simulink model "dynamic_model_v4"  (R2022a)
settings: Solver=VariableStepAuto  StartTime=0.0  StopTime=T  FixedStep=0.001  RelTol=1e-3  AbsTol=1e-3  EnableMultiTasking=on
values from neighbouring files (symbols this model uses):
  Kv = 1*(ones(3,3))    [RBT_UR5_NN_adaptation.m]    (also in dynamic_model_code.m = [1.5, 0, 0)
  lamda = 0.1    [RBT_UR5_NN_adaptation.m]    (also in dynamic_model_code.m = 1.2)
  M = A1*layer1    [M_cap.m]    (also in dynamic_model_code.m = 5)
  m1 = 1    [dynamic_model_code.m]
  m2 = 0.5    [dynamic_model_code.m]
  m3 = 0.25    [dynamic_model_code.m]
  s = tf('s')    [tf_compute.m]
  w = zeros(3,1)    [RBT_UR5_NN_adaptation.m]    (also in dynamic_model_code.m)
undefined symbols (not defined in the file or in its folder): X, Y, Z
libraries: sm_lib x15, nesl_utility x13, simulink x9
settings Model: Creator=khan  LastModifiedBy=khan
settings SolverCC: AutoScaleAbsTol=off  AlgebraicLoopSolver=TrustRegion  MaxZcPerStep=1
settings DataIOCC: LimitDataPoints=on  MaxDataPoints=10000
settings OptimizationCC: LifeSpan=inf
settings DebuggingCC: UnconnectedInputMsg=warning  UnconnectedOutputMsg=warning  UnconnectedLineMsg=warning  AllowSymbolicDim=off  SFUnexpectedBacktrackingDiag=warning  SFNoUnconditionalDefaultTransitionDiag=warning  SFExecutionAtInitializationDiag=none  SFMachineParentedDataDiag=warning  ArithmeticOperatorsInVariantConditions=warning
settings SFSimCC: SimUseLocalCustomCode=off  CustomCodeUndefinedFunction=UseInterfaceOnly
settings RTWCC: RTWUseLocalCustomCode=off  DLArmComputeVersion=19.05
settings CodeAppCC: StateflowObjectComments=on
settings GRTTargetCC: TargetLangStandard=C89/C90 (ANSI)
settings ConfigComp: CovMetricSettings=dw  CovSaveCumulativeToWorkspaceVar=on  CovSaveSingleToWorkspaceVar=on  CovExternalEMLEnable=off  CovSFcnEnable=off
settings SimscapeCC: SimscapeLogType=all  SimscapeLogSimulationStatistics=on  SimscapeLogDataHistory=10000

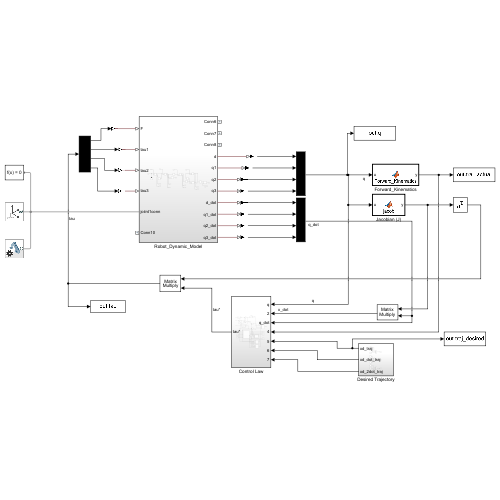
[thumbnail: Simulink's stored preview of the top-level diagram]
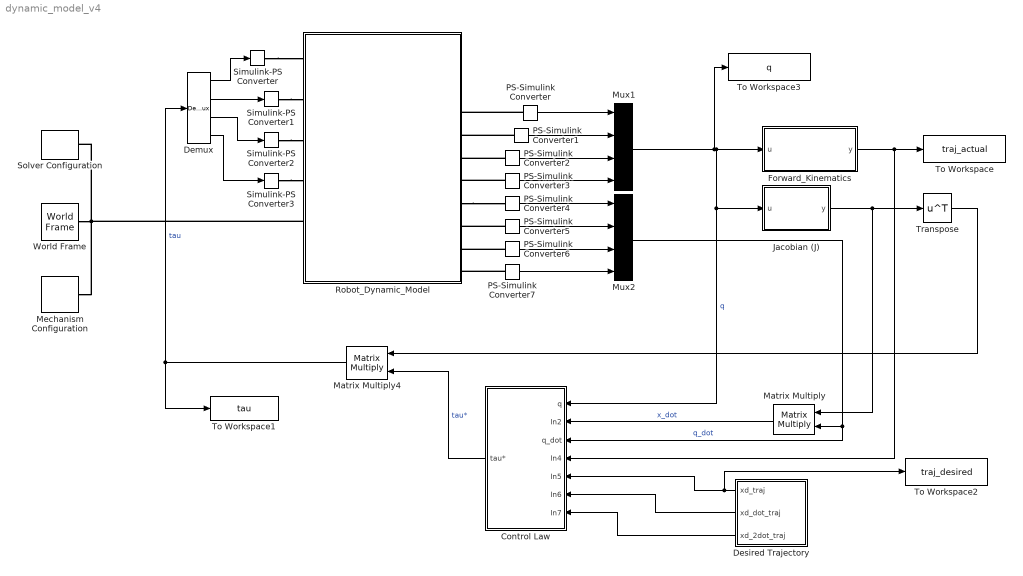
== system dynamic_model_v4 ==
  Control Law : Subsystem
  Demux : Demux
  Desired Trajectory : Subsystem
  Forward_Kinematics : MATLAB Function  TreatAsAtomicUnit=on
  Jacobian (J) : MATLAB Function  TreatAsAtomicUnit=on
  Matrix Multiply : Product  Multiplication=Matrix(*)
  Matrix Multiply4 : Product  Multiplication=Matrix(*)
  Mechanism Configuration : sm_lib/Utilities/Mechanism Configuration  UniformGravity=Constant  GravityVector=[0 0 -9.80665]  GravityUnits=m/s^2  LinearizationDelta=0.001  JointModeTransitionNonlinearIterations=2
  Mux1 : Mux
  Mux2 : Mux
  PS-Simulink Converter{,1..7} (8 alike) : nesl_utility/PS-Simulink Converter  PhysicalDomain=network_engine_domain  SubClassName=ps_output  LeftPortType=input  RightPortType=output  PseudoPeriodic=off  Frequencies=[]  VectorFormat=inherit  Unit=inherit  AffineConversion=off
      settings: SourceProductBaseCode=SS,PW,VE
  Robot_Dynamic_Model : Subsystem
  Simulink-PS Converter : nesl_utility/Simulink-PS Converter  PhysicalDomain=network_engine_domain  SubClassName=ps_input  LeftPortType=input  RightPortType=output  PseudoPeriodic=off  Frequencies=[]  NoiseDistribution=none  NoiseParameters=[]  Unit=N  AffineConversion=off  FilteringAndDerivatives=provide  SimscapeFilterOrder=1  InputFilterTimeConstant=0.001  UdotUserProvided=0
      settings: SourceProductBaseCode=SS,PW,VE
  Simulink-PS Converter1 : nesl_utility/Simulink-PS Converter  PhysicalDomain=network_engine_domain  SubClassName=ps_input  LeftPortType=input  RightPortType=output  PseudoPeriodic=off  Frequencies=[]  NoiseDistribution=none  NoiseParameters=[]  Unit=N*m  AffineConversion=off  FilteringAndDerivatives=provide  SimscapeFilterOrder=1  InputFilterTimeConstant=0.001  UdotUserProvided=0
      settings: SourceProductBaseCode=SS,PW,VE
  Simulink-PS Converter2 : nesl_utility/Simulink-PS Converter  PhysicalDomain=network_engine_domain  SubClassName=ps_input  LeftPortType=input  RightPortType=output  PseudoPeriodic=off  Frequencies=[]  NoiseDistribution=none  NoiseParameters=[]  Unit=N*m  AffineConversion=off  FilteringAndDerivatives=provide  SimscapeFilterOrder=1  InputFilterTimeConstant=0.001  UdotUserProvided=0
      settings: SourceProductBaseCode=SS,PW,VE
  Simulink-PS Converter3 : nesl_utility/Simulink-PS Converter  PhysicalDomain=network_engine_domain  SubClassName=ps_input  LeftPortType=input  RightPortType=output  PseudoPeriodic=off  Frequencies=[]  NoiseDistribution=none  NoiseParameters=[]  Unit=N*m  AffineConversion=off  FilteringAndDerivatives=provide  SimscapeFilterOrder=1  InputFilterTimeConstant=0.001  UdotUserProvided=0
      settings: SourceProductBaseCode=SS,PW,VE
  Solver Configuration : nesl_utility/Solver Configuration  PhysicalDomain=network_engine_domain  SubClassName=solver  LeftPortType=input  RightPortType=generic  Tones=[]  Harmonics=[]  SimulateNoise=off  Profile=off  UseLocalSampling=off  EnableSwitchedLinearOptims=on  FrequencyDomain=off  UseCCode=off  RelTol=0.001  AbsTol=1e-06  MinStep=1e-09  ToWorkspace=off  RevertToSquareIcSolve=off  NumHomotopyIterations=100  PhasorMode=off  PhasorModeNumHarmonics=1  IndexReductionMethod=DerivativeReplacement  DoDC=off  ResidualTolerance=1e-09  UseLocalSolver=off  LocalSolverChoice=NE_BACKWARD_EULER_ADVANCER  LocalSolverSampleTime=0.001  DoFixedCost=off  MaxNonlinIter=3  MaxModeIter=2  ComputeImpulses=off  ImpulseIterations=2  LinearAlgebra=Sparse  LinearAlgebraNumThread=0  EquationFormulation=NE_TIME_EF  DelaysMemoryBudget=1024  AutomaticFiltering=on  FilteringTimeConstant=0.001  PartitionStorageMethod=AS_NEEDED  PartitionMemoryBudget=1024  PartitionMethod=FAST
      settings: SourceProductBaseCode=SS,PW,VE
  To Workspace : ToWorkspace  VariableName=traj_actual  SampleTime=-1
  To Workspace1 : ToWorkspace  VariableName=tau  SampleTime=-1
      settings: Save2DSignal=2-D array (concatenate along first dimension)
  To Workspace2 : ToWorkspace  VariableName=traj_desired  SampleTime=-1
  To Workspace3 : ToWorkspace  VariableName=q  SampleTime=-1
  Transpose : Math  Operator=transpose
  World Frame : sm_lib/Frames and Transforms/World Frame
  wires:
  Forward_Kinematics/1(y) -> Control Law/4(In4), To Workspace/1
  PS-Simulink Converter/1 -> Mux1/1
  PS-Simulink Converter1/1 -> Mux1/2
  PS-Simulink Converter2/1 -> Mux1/3
  PS-Simulink Converter3/1 -> Mux1/4
  PS-Simulink Converter4/1 -> Mux2/1
  PS-Simulink Converter5/1 -> Mux2/2
  PS-Simulink Converter6/1 -> Mux2/3
  PS-Simulink Converter7/1 -> Mux2/4
  Jacobian (J)/1(y) -> Matrix Multiply/1, Transpose/1
  Transpose/1 -> Matrix Multiply4/1
  Matrix Multiply4/1 -> Demux/1, To Workspace1/1  "tau"
  Demux/1 -> Simulink-PS Converter/1
  Demux/2 -> Simulink-PS Converter1/1
  Demux/3 -> Simulink-PS Converter2/1
  Demux/4 -> Simulink-PS Converter3/1
  Matrix Multiply/1 -> Control Law/2(In2)  "x_dot"
  Desired Trajectory/1(xd_traj) -> To Workspace2/1, Control Law/5(In5)
  Desired Trajectory/2(xd_dot_traj) -> Control Law/6(In6)
  Desired Trajectory/3(xd_2dot_traj) -> Control Law/7(In7)
  Control Law/1(tau*) -> Matrix Multiply4/2  "tau*"
  Mux1/1 -> Forward_Kinematics/1(u), Control Law/1(q), Jacobian (J)/1(u), To Workspace3/1  "q"
  Mux2/1 -> Matrix Multiply/2, Control Law/3(q_dot)  "q_dot"
  connections:
  World Frame/RConn1 -- Mechanism Configuration/RConn1 -- Robot_Dynamic_Model/LConn5 -- Solver Configuration/RConn1
  PS-Simulink Converter/LConn1 -- Robot_Dynamic_Model/RConn4
  PS-Simulink Converter1/LConn1 -- Robot_Dynamic_Model/RConn5
  PS-Simulink Converter2/LConn1 -- Robot_Dynamic_Model/RConn6
  PS-Simulink Converter3/LConn1 -- Robot_Dynamic_Model/RConn7
  Robot_Dynamic_Model/RConn8 -- PS-Simulink Converter4/LConn1
  PS-Simulink Converter5/LConn1 -- Robot_Dynamic_Model/RConn9
  PS-Simulink Converter6/LConn1 -- Robot_Dynamic_Model/RConn10
  PS-Simulink Converter7/LConn1 -- Robot_Dynamic_Model/RConn11
  Simulink-PS Converter/RConn1 -- Robot_Dynamic_Model/LConn1
  Simulink-PS Converter1/RConn1 -- Robot_Dynamic_Model/LConn2
  Simulink-PS Converter2/RConn1 -- Robot_Dynamic_Model/LConn3
  Simulink-PS Converter3/RConn1 -- Robot_Dynamic_Model/LConn4

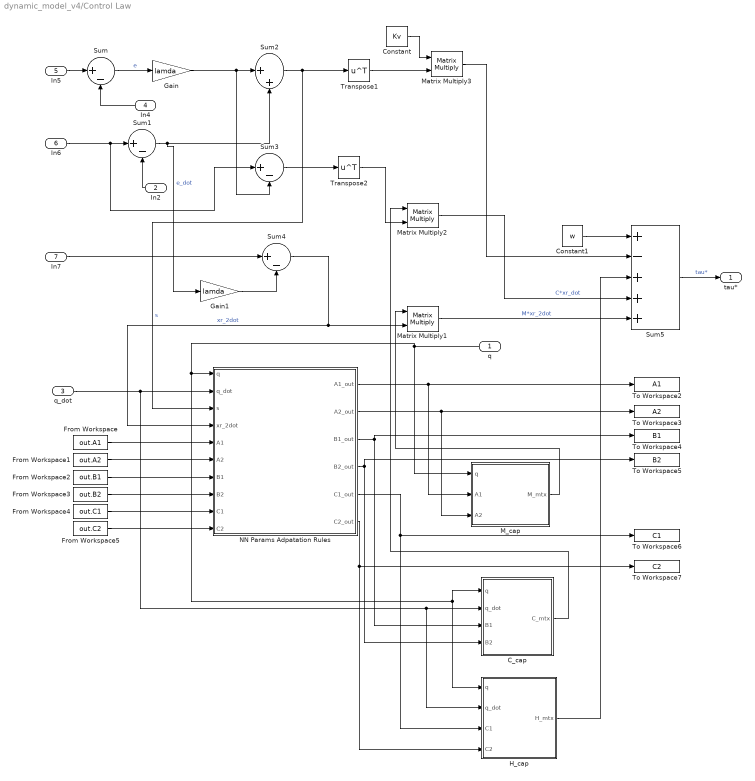
== system dynamic_model_v4/Control Law ==
  q : Inport
  In2 : Inport  Port=2
  q_dot : Inport  Port=3
  In4 : Inport  Port=4
  In5 : Inport  Port=5
  In6 : Inport  Port=6
  In7 : Inport  Port=7
  C_cap : MATLAB Function  TreatAsAtomicUnit=on
  Constant : Constant  Value=Kv
  Constant1 : Constant  Value=w
  From Workspace : FromWorkspace  VariableName=out.A1
  From Workspace1 : FromWorkspace  VariableName=out.A2
  From Workspace2 : FromWorkspace  VariableName=out.B1
  From Workspace3 : FromWorkspace  VariableName=out.B2
  From Workspace4 : FromWorkspace  VariableName=out.C1
  From Workspace5 : FromWorkspace  VariableName=out.C2
  Gain : Gain  Gain=lamda
  Gain1 : Gain  Gain=lamda
  H_cap : MATLAB Function  TreatAsAtomicUnit=on
  M_cap : MATLAB Function  TreatAsAtomicUnit=on
  Matrix Multiply1 : Product  Multiplication=Matrix(*)
  Matrix Multiply2 : Product  Multiplication=Matrix(*)
  Matrix Multiply3 : Product  Multiplication=Matrix(*)
  NN Params Adpatation Rules : MATLAB Function  TreatAsAtomicUnit=on
  Sum{,1,3..4} (4 alike) : Sum  Inputs=|+-
  Sum2 : Sum  Inputs=|++
  Sum5 : Sum  Inputs=+-+++
  To Workspace2 : ToWorkspace  VariableName=A1  SaveFormat=Timeseries  SampleTime=-1
  To Workspace3 : ToWorkspace  VariableName=A2  SaveFormat=Timeseries  SampleTime=-1
  To Workspace4 : ToWorkspace  VariableName=B1  SaveFormat=Timeseries  SampleTime=-1
  To Workspace5 : ToWorkspace  VariableName=B2  SaveFormat=Timeseries  SampleTime=-1
  To Workspace6 : ToWorkspace  VariableName=C1  SaveFormat=Timeseries  SampleTime=-1
  To Workspace7 : ToWorkspace  VariableName=C2  SaveFormat=Timeseries  SampleTime=-1
  Transpose1 : Math  Operator=transpose
  Transpose2 : Math  Operator=transpose
  tau* : Outport
  wires:
  From Workspace2/1 -> NN Params Adpatation Rules/7(B1)
  Matrix Multiply1/1 -> Sum5/5  "M*xr_2dot"
  NN Params Adpatation Rules/3(B1_out) -> C_cap/3(B1), To Workspace4/1
  q_dot/1 -> NN Params Adpatation Rules/2(q_dot), H_cap/2(q_dot), C_cap/2(q_dot)
  NN Params Adpatation Rules/4(B2_out) -> To Workspace5/1, C_cap/4(B2)
  From Workspace1/1 -> NN Params Adpatation Rules/6(A2)
  NN Params Adpatation Rules/2(A2_out) -> M_cap/3(A2), To Workspace3/1
  Sum3/1 -> Transpose2/1
  Sum5/1 -> tau*/1  "tau*"
  Sum/1 -> Gain/1  "e"
  Gain/1 -> Sum2/1, Sum3/2
  Constant/1 -> Matrix Multiply3/1
  Sum1/1 -> Gain1/1, Sum2/2  "e_dot"
  C_cap/1(C_mtx) -> Matrix Multiply2/1
  From Workspace/1 -> NN Params Adpatation Rules/5(A1)
  NN Params Adpatation Rules/5(C1_out) -> H_cap/3(C1), To Workspace6/1
  NN Params Adpatation Rules/6(C2_out) -> To Workspace7/1, H_cap/4(C2)
  NN Params Adpatation Rules/1(A1_out) -> To Workspace2/1, M_cap/2(A1)
  q/1 -> M_cap/1(q), NN Params Adpatation Rules/1(q), H_cap/1(q), C_cap/1(q)
  Transpose1/1 -> Matrix Multiply3/2
  Sum4/1 -> NN Params Adpatation Rules/4(xr_2dot), Matrix Multiply1/2  "xr_2dot"
  In5/1 -> Sum/1
  In6/1 -> Sum3/1, Sum1/1
  From Workspace4/1 -> NN Params Adpatation Rules/9(C1)
  Constant1/1 -> Sum5/1
  Sum2/1 -> Transpose1/1, NN Params Adpatation Rules/3(s)  "s"
  From Workspace3/1 -> NN Params Adpatation Rules/8(B2)
  Transpose2/1 -> Matrix Multiply2/2
  H_cap/1(H_mtx) -> Sum5/3
  M_cap/1(M_mtx) -> Matrix Multiply1/1
  Gain1/1 -> Sum4/2
  Matrix Multiply3/1 -> Sum5/2
  Matrix Multiply2/1 -> Sum5/4  "C*xr_dot"
  From Workspace5/1 -> NN Params Adpatation Rules/10(C2)
  In7/1 -> Sum4/1
  In4/1 -> Sum/2
  In2/1 -> Sum1/2

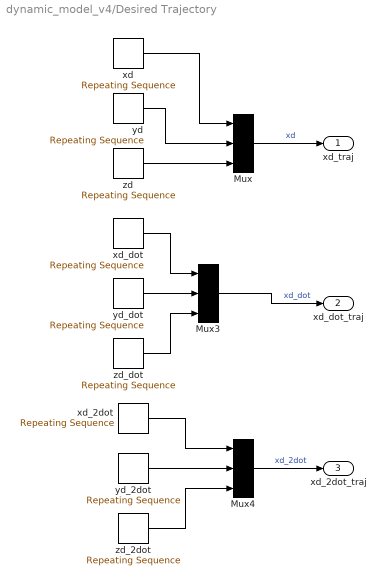
== system dynamic_model_v4/Desired Trajectory ==
  Mux : Mux  Inputs=3
  Mux3 : Mux  Inputs=3
  Mux4 : Mux  Inputs=3
  xd : simulink/Sources/Repeating Sequence  rep_seq_t=t  rep_seq_y=px
  xd_2dot : simulink/Sources/Repeating Sequence  rep_seq_t=t  rep_seq_y=ax
  xd_dot : simulink/Sources/Repeating Sequence  rep_seq_t=t  rep_seq_y=vx
  yd : simulink/Sources/Repeating Sequence  rep_seq_t=t  rep_seq_y=py
  yd_2dot : simulink/Sources/Repeating Sequence  rep_seq_t=t  rep_seq_y=ay
  yd_dot : simulink/Sources/Repeating Sequence  rep_seq_t=t  rep_seq_y=vy
  zd : simulink/Sources/Repeating Sequence  rep_seq_t=t  rep_seq_y=pz
  zd_2dot : simulink/Sources/Repeating Sequence  rep_seq_t=t  rep_seq_y=az
  zd_dot : simulink/Sources/Repeating Sequence  rep_seq_t=t  rep_seq_y=vz
  xd_traj : Outport
  xd_dot_traj : Outport  Port=2
  xd_2dot_traj : Outport  Port=3
  wires:
  zd_dot/1 -> Mux3/3
  yd_dot/1 -> Mux3/2
  zd/1 -> Mux/3
  xd_2dot/1 -> Mux4/1
  yd/1 -> Mux/2
  xd_dot/1 -> Mux3/1
  yd_2dot/1 -> Mux4/2
  zd_2dot/1 -> Mux4/3
  Mux3/1 -> xd_dot_traj/1  "xd_dot"
  xd/1 -> Mux/1
  Mux4/1 -> xd_2dot_traj/1  "xd_2dot"
  Mux/1 -> xd_traj/1  "xd"

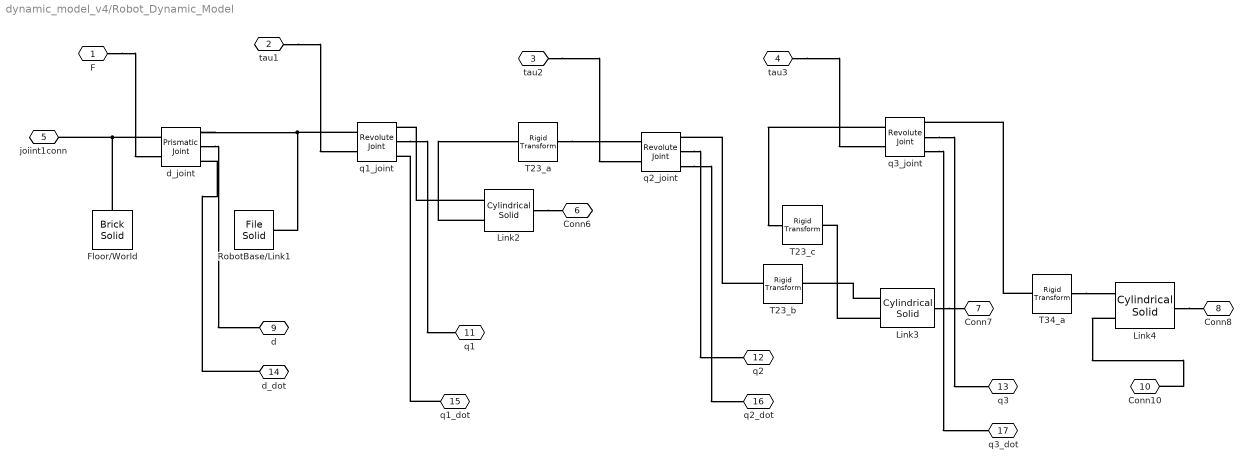
== system dynamic_model_v4/Robot_Dynamic_Model ==
  Floor/World : sm_lib/Body Elements/Brick Solid  GraphicAmbientColor=[0.15 0.15 0.15 1.0]  BasedOnType=Density  BrickDimensions=[340 220 10]  BrickDimensionUnits=mm  CenterOfMass=[0 0 0]  CenterOfMassUnits=m  GraphicDiffuseColor=[0.5 0.5 0.5]  Density=1000  DensityUnits=kg/m^3  DoExposeReferenceFrame=on  GraphicEmissiveColor=[0.0 0.0 0.0 1.0]  ExportEntireGeometry=off  SerializedFrames=<Frames/>  MarkerShape=Sphere  MarkerSize=10  GraphicType=FromGeometry  InertiaType=CalculateFromGeometry  Mass=1  MassUnits=kg  MomentsOfInertia=[1 1 1]  MomentsOfInertiaUnits=kg*m^2  GraphicOpacity=1.0  ProductsOfInertia=[0 0 0]  ProductsOfInertiaUnits=kg*m^2  GraphicShininess=75  GraphicSpecularColor=[0.5 0.5 0.5 1.0]  GraphicVisPropType=SimpleVisualProperties
  Link2 : sm_lib/Body Elements/Cylindrical Solid  GraphicAmbientColor=[0.15 0.15 0.15 1.0]  BasedOnType=Mass  CenterOfMass=[0 0 0]  CenterOfMassUnits=m  GraphicDiffuseColor=[0.5 0.0 0.0]  CylinderLength=L1  CylinderLengthUnits=m  CylinderRadius=25  CylinderRadiusUnits=mm  Density=1000  DensityUnits=kg/m^3  DoExposeReferenceFrame=on  GraphicEmissiveColor=[0.0 0.0 0.0 1.0]  ExportEntireGeometry=off  SerializedFrames=<Frames><Frame><Id>Frame1</Id><Value><Name>bot</Name><Origin><Source>GeometricFeature</Source><FeatureName>bottom surface</FeatureName></Origin><PrimaryAxis><DefinedDirection>+Z</DefinedDirection><Source>ReferenceFrame</Source><SourceDirection>+Z</SourceDirection><FeatureName></FeatureName></PrimaryAxis><SecondaryAxis><DefinedDirection>+X</DefinedDirection><Source>ReferenceFrame</Source><SourceDirection>+X</SourceDirection><FeatureName></FeatureName></SecondaryAxis></Value></Frame><Frame><Id>Frame2</Id><Value><Name>top</Name><Origin><Source>GeometricFeature</Source><FeatureName>top surface</FeatureName></Origin><PrimaryAxis><DefinedDirection>+Z</DefinedDirection><Source>ReferenceFrame</Source><SourceDirection>+Z</SourceDirection><FeatureName></FeatureName></PrimaryAxis><SecondaryAxis><DefinedDirection>+X</DefinedDirection><Source>ReferenceFrame</Source><SourceDirection>+X</SourceDirection><FeatureName></FeatureName></SecondaryAxis></Value></Frame></Frames>  MarkerShape=Sphere  MarkerSize=10  GraphicType=FromGeometry  InertiaType=CalculateFromGeometry  Mass=m1  MassUnits=kg  MomentsOfInertia=[1 1 1]  MomentsOfInertiaUnits=kg*m^2  GraphicOpacity=1.0  ProductsOfInertia=[0 0 0]  ProductsOfInertiaUnits=kg*m^2  GraphicShininess=75  GraphicSpecularColor=[0.5 0.5 0.5 1.0]  GraphicVisPropType=AdvancedVisualProperties
  Link3 : sm_lib/Body Elements/Cylindrical Solid  GraphicAmbientColor=[0.15 0.15 0.15 1.0]  BasedOnType=Mass  CenterOfMass=[0 0 0]  CenterOfMassUnits=m  GraphicDiffuseColor=[0.0 0.0 1.0]  CylinderLength=L2  CylinderLengthUnits=m  CylinderRadius=25  CylinderRadiusUnits=mm  Density=1000  DensityUnits=kg/m^3  DoExposeReferenceFrame=on  GraphicEmissiveColor=[0.0 0.0 0.0 1.0]  ExportEntireGeometry=off  SerializedFrames=<Frames><Frame><Id>Frame1</Id><Value><Name>bot</Name><Origin><Source>GeometricFeature</Source><FeatureName>bottom surface</FeatureName></Origin><PrimaryAxis><DefinedDirection>+Z</DefinedDirection><Source>ReferenceFrame</Source><SourceDirection>+Z</SourceDirection><FeatureName></FeatureName></PrimaryAxis><SecondaryAxis><DefinedDirection>+X</DefinedDirection><Source>ReferenceFrame</Source><SourceDirection>+X</SourceDirection><FeatureName></FeatureName></SecondaryAxis></Value></Frame><Frame><Id>Frame2</Id><Value><Name>top</Name><Origin><Source>GeometricFeature</Source><FeatureName>top surface</FeatureName></Origin><PrimaryAxis><DefinedDirection>+Z</DefinedDirection><Source>ReferenceFrame</Source><SourceDirection>+Z</SourceDirection><FeatureName></FeatureName></PrimaryAxis><SecondaryAxis><DefinedDirection>+X</DefinedDirection><Source>ReferenceFrame</Source><SourceDirection>+X</SourceDirection><FeatureName></FeatureName></SecondaryAxis></Value></Frame></Frames>  MarkerShape=Sphere  MarkerSize=10  GraphicType=FromGeometry  InertiaType=CalculateFromGeometry  Mass=m2  MassUnits=kg  MomentsOfInertia=[1 1 1]  MomentsOfInertiaUnits=kg*m^2  GraphicOpacity=1.0  ProductsOfInertia=[0 0 0]  ProductsOfInertiaUnits=kg*m^2  GraphicShininess=75  GraphicSpecularColor=[0.5 0.5 0.5 1.0]  GraphicVisPropType=SimpleVisualProperties
  Link4 : sm_lib/Body Elements/Cylindrical Solid  GraphicAmbientColor=[0.15 0.15 0.15 1.0]  BasedOnType=Mass  CenterOfMass=[0 0 0]  CenterOfMassUnits=m  GraphicDiffuseColor=[0.0 1.0 0.0]  CylinderLength=L3  CylinderLengthUnits=m  CylinderRadius=25  CylinderRadiusUnits=mm  Density=1000  DensityUnits=kg/m^3  DoExposeReferenceFrame=on  GraphicEmissiveColor=[0.0 0.0 0.0 1.0]  ExportEntireGeometry=off  SerializedFrames=<Frames><Frame><Id>Frame1</Id><Value><Name>bot</Name><Origin><Source>GeometricFeature</Source><FeatureName>bottom surface</FeatureName></Origin><PrimaryAxis><DefinedDirection>+Z</DefinedDirection><Source>ReferenceFrame</Source><SourceDirection>+Z</SourceDirection><FeatureName></FeatureName></PrimaryAxis><SecondaryAxis><DefinedDirection>+X</DefinedDirection><Source>ReferenceFrame</Source><SourceDirection>+X</SourceDirection><FeatureName></FeatureName></SecondaryAxis></Value></Frame><Frame><Id>Frame2</Id><Value><Name>top</Name><Origin><Source>GeometricFeature</Source><FeatureName>top surface</FeatureName></Origin><PrimaryAxis><DefinedDirection>+Z</DefinedDirection><Source>ReferenceFrame</Source><SourceDirection>+Z</SourceDirection><FeatureName></FeatureName></PrimaryAxis><SecondaryAxis><DefinedDirection>+X</DefinedDirection><Source>ReferenceFrame</Source><SourceDirection>+X</SourceDirection><FeatureName></FeatureName></SecondaryAxis></Value></Frame></Frames>  MarkerShape=Sphere  MarkerSize=10  GraphicType=FromGeometry  InertiaType=CalculateFromGeometry  Mass=m3  MassUnits=kg  MomentsOfInertia=[1 1 1]  MomentsOfInertiaUnits=kg*m^2  GraphicOpacity=1.0  ProductsOfInertia=[0 0 0]  ProductsOfInertiaUnits=kg*m^2  GraphicShininess=75  GraphicSpecularColor=[0.5 0.5 0.5 1.0]  GraphicVisPropType=SimpleVisualProperties
  RobotBase/Link1 : sm_lib/Body Elements/File Solid  ExtGeomFileName=D:\Graduate\CourseWork\Sem4_Winter2023\AdaptiveControl\Project\CADfiles\robot_base.STEP  UnitType=Custom  ExtGeomFileUnits=mm  StepReaderType=HEX  ExportConvexHullGeometry=off  InertiaType=CalculateFromGeometry  Mass=M  MassUnits=kg  CenterOfMass=[0 0 0]  CenterOfMassUnits=m  MomentsOfInertia=[1 1 1]  MomentsOfInertiaUnits=kg*m^2  ProductsOfInertia=[0 0 0]  ProductsOfInertiaUnits=kg*m^2  BasedOnType=Mass  Density=1000  DensityUnits=kg/m^3  DoExposeReferenceFrame=on  SerializedFrames=<Frames/>  GraphicType=FromGeometry  MarkerShape=Sphere  MarkerSize=10  GraphicVisPropType=SimpleVisualProperties  GraphicDiffuseColor=[0.5 0.5 0.5]  GraphicSpecularColor=[0.5 0.5 0.5 1.0]  GraphicAmbientColor=[0.15 0.15 0.15 1.0]  GraphicEmissiveColor=[0.0 0.0 0.0 1.0]  GraphicShininess=75  GraphicOpacity=1.0
  T23_a : sm_lib/Frames and Transforms/Rigid Transform  TranslationMethod=None  TranslationStandardOffset=0  TranslationLengthUnit=m  TranslationStandardAxis=+Z  TranslationCartesianOffset=[0 0 0]  TranslationROffset=0  TranslationROffsetUnits=m  TranslationZOffset=0  TranslationZOffsetUnits=m  TranslationThetaOffset=0  TranslationThetaOffsetUnits=deg  RotationMethod=StandardAxis  RotationAngleUnits=deg  RotationStandardAxis=+X  RotationAngle=90.0  RotationArbitraryAxis=[0 0 1]  FollAlignAxisA=+X  BaseAlignAxisA=+Y  FollAlignAxisB=+Y  BaseAlignAxisB=+Z  RotationSequenceAxes=FollowerAxes  RotationSequence=XZY  RotationSequenceAngles=[90 -90 0]  RotationSequenceAnglesUnits=deg  RotationMatrix=[1 0 0; 0 1 0; 0 0 1]
  T23_b : sm_lib/Frames and Transforms/Rigid Transform  TranslationMethod=None  TranslationStandardOffset=0  TranslationLengthUnit=m  TranslationStandardAxis=+Z  TranslationCartesianOffset=[0 0 0]  TranslationROffset=0  TranslationROffsetUnits=m  TranslationZOffset=0  TranslationZOffsetUnits=m  TranslationThetaOffset=0  TranslationThetaOffsetUnits=deg  RotationMethod=RotationSequence  RotationAngleUnits=deg  RotationStandardAxis=+X  RotationAngle=90.0  RotationArbitraryAxis=[0 0 1]  FollAlignAxisA=+X  BaseAlignAxisA=+Y  FollAlignAxisB=+Y  BaseAlignAxisB=+Z  RotationSequenceAxes=FollowerAxes  RotationSequence=XZY  RotationSequenceAngles=[90 90 0]  RotationSequenceAnglesUnits=deg  RotationMatrix=[1 0 0; 0 1 0; 0 0 1]
  T23_c : sm_lib/Frames and Transforms/Rigid Transform  TranslationMethod=None  TranslationStandardOffset=0  TranslationLengthUnit=m  TranslationStandardAxis=+Z  TranslationCartesianOffset=[0 0 0]  TranslationROffset=0  TranslationROffsetUnits=m  TranslationZOffset=0  TranslationZOffsetUnits=m  TranslationThetaOffset=0  TranslationThetaOffsetUnits=deg  RotationMethod=RotationSequence  RotationAngleUnits=deg  RotationStandardAxis=+X  RotationAngle=90.0  RotationArbitraryAxis=[0 0 1]  FollAlignAxisA=+X  BaseAlignAxisA=+Y  FollAlignAxisB=+Y  BaseAlignAxisB=+Z  RotationSequenceAxes=FollowerAxes  RotationSequence=XZY  RotationSequenceAngles=[90 90 0]  RotationSequenceAnglesUnits=deg  RotationMatrix=[1 0 0; 0 1 0; 0 0 1]
  T34_a : sm_lib/Frames and Transforms/Rigid Transform  TranslationMethod=None  TranslationStandardOffset=0  TranslationLengthUnit=m  TranslationStandardAxis=+Z  TranslationCartesianOffset=[0 0 0]  TranslationROffset=0  TranslationROffsetUnits=m  TranslationZOffset=0  TranslationZOffsetUnits=m  TranslationThetaOffset=0  TranslationThetaOffsetUnits=deg  RotationMethod=RotationSequence  RotationAngleUnits=deg  RotationStandardAxis=+X  RotationAngle=90.0  RotationArbitraryAxis=[0 0 1]  FollAlignAxisA=+X  BaseAlignAxisA=+Y  FollAlignAxisB=+Y  BaseAlignAxisB=+Z  RotationSequenceAxes=FollowerAxes  RotationSequence=XZY  RotationSequenceAngles=[90 90 0]  RotationSequenceAnglesUnits=deg  RotationMatrix=[1 0 0; 0 1 0; 0 0 1]
  d_joint : sm_lib/Joints/Prismatic Joint  JointMode=Normal  SenseConstraintForce=off  SenseConstraintForceX=off  SenseConstraintForceY=off  SenseConstraintForceZ=off  SenseConstraintTorque=off  SenseConstraintTorqueX=off  SenseConstraintTorqueY=off  SenseConstraintTorqueZ=off  SenseTotalForce=off  SenseTotalForceX=off  SenseTotalForceY=off  SenseTotalForceZ=off  SenseTotalTorque=off  SenseTotalTorqueX=off  SenseTotalTorqueY=off  SenseTotalTorqueZ=off  CompositeWrenchDir=FollowerOnBase  CompositeWrenchFrame=BaseFrame  EquilibriumPosition=0  EquilibriumPositionUnits=m  SpringStiffness=0  SpringStiffnessUnits=N/m  DampingCoefficient=B  DampingCoefficientUnits=N/(m/s)  TorqueActuationMode=InputTorque  MotionActuationMode=ComputedMotion  SensePosition=on  SenseVelocity=on  SenseAcceleration=off  SenseTorqueForce=off  SenseLowerLimitTorqueForce=off  SenseUpperLimitTorqueForce=off  LowerLimitSpecify=on  LowerLimitBound=0  LowerLimitBoundUnits=m  LowerLimitStiffness=1e6  LowerLimitStiffnessUnits=N/m  LowerLimitDamping=1e3  LowerLimitDampingUnits=N/(m/s)  LowerLimitTransitionRegionWidth=1e-4  LowerLimitTransitionRegionWidthUnits=m  UpperLimitSpecify=on  UpperLimitBound=0.254  UpperLimitBoundUnits=m  UpperLimitStiffness=1e6  UpperLimitStiffnessUnits=N/m  UpperLimitDamping=1e3  UpperLimitDampingUnits=N/(m/s)  UpperLimitTransitionRegionWidth=1e-4  UpperLimitTransitionRegionWidthUnits=m  PositionTargetSpecify=off  PositionTargetPriority=High  PositionTargetValue=0  PositionTargetValueUnits=m  VelocityTargetSpecify=off  VelocityTargetPriority=High  VelocityTargetValue=0  VelocityTargetValueUnits=m/s
  q1_joint : sm_lib/Joints/Revolute Joint  JointMode=Normal  SenseConstraintForce=off  SenseConstraintForceX=off  SenseConstraintForceY=off  SenseConstraintForceZ=off  SenseConstraintTorque=off  SenseConstraintTorqueX=off  SenseConstraintTorqueY=off  SenseConstraintTorqueZ=off  SenseTotalForce=off  SenseTotalForceX=off  SenseTotalForceY=off  SenseTotalForceZ=off  SenseTotalTorque=off  SenseTotalTorqueX=off  SenseTotalTorqueY=off  SenseTotalTorqueZ=off  CompositeWrenchDir=FollowerOnBase  CompositeWrenchFrame=BaseFrame  EquilibriumPosition=0  EquilibriumPositionUnits=deg  SpringStiffness=0  SpringStiffnessUnits=N*m/deg  DampingCoefficient=b1  DampingCoefficientUnits=N*m/(deg/s)  TorqueActuationMode=InputTorque  MotionActuationMode=ComputedMotion  SensePosition=on  SenseVelocity=on  SenseAcceleration=off  SenseTorqueForce=off  SenseLowerLimitTorqueForce=off  SenseUpperLimitTorqueForce=off  LowerLimitSpecify=off  LowerLimitBound=0  LowerLimitBoundUnits=deg  LowerLimitStiffness=1e4  LowerLimitStiffnessUnits=N*m/deg  LowerLimitDamping=10  LowerLimitDampingUnits=N*m/(deg/s)  LowerLimitTransitionRegionWidth=0.1  LowerLimitTransitionRegionWidthUnits=deg  UpperLimitSpecify=off  UpperLimitBound=10  UpperLimitBoundUnits=deg  UpperLimitStiffness=1e4  UpperLimitStiffnessUnits=N*m/deg  UpperLimitDamping=10  UpperLimitDampingUnits=N*m/(deg/s)  UpperLimitTransitionRegionWidth=0.1  UpperLimitTransitionRegionWidthUnits=deg  PositionTargetSpecify=off  PositionTargetPriority=High  PositionTargetValue=0  PositionTargetValueUnits=deg  VelocityTargetSpecify=off  VelocityTargetPriority=High  VelocityTargetValue=0  VelocityTargetValueUnits=deg/s
  q2_joint : sm_lib/Joints/Revolute Joint  JointMode=Normal  SenseConstraintForce=off  SenseConstraintForceX=off  SenseConstraintForceY=off  SenseConstraintForceZ=off  SenseConstraintTorque=off  SenseConstraintTorqueX=off  SenseConstraintTorqueY=off  SenseConstraintTorqueZ=off  SenseTotalForce=off  SenseTotalForceX=off  SenseTotalForceY=off  SenseTotalForceZ=off  SenseTotalTorque=off  SenseTotalTorqueX=off  SenseTotalTorqueY=off  SenseTotalTorqueZ=off  CompositeWrenchDir=FollowerOnBase  CompositeWrenchFrame=BaseFrame  EquilibriumPosition=0  EquilibriumPositionUnits=deg  SpringStiffness=0  SpringStiffnessUnits=N*m/deg  DampingCoefficient=b2  DampingCoefficientUnits=N*m/(deg/s)  TorqueActuationMode=InputTorque  MotionActuationMode=ComputedMotion  SensePosition=on  SenseVelocity=on  SenseAcceleration=off  SenseTorqueForce=off  SenseLowerLimitTorqueForce=off  SenseUpperLimitTorqueForce=off  LowerLimitSpecify=off  LowerLimitBound=0  LowerLimitBoundUnits=deg  LowerLimitStiffness=1e4  LowerLimitStiffnessUnits=N*m/deg  LowerLimitDamping=10  LowerLimitDampingUnits=N*m/(deg/s)  LowerLimitTransitionRegionWidth=0.1  LowerLimitTransitionRegionWidthUnits=deg  UpperLimitSpecify=off  UpperLimitBound=360  UpperLimitBoundUnits=deg  UpperLimitStiffness=1e4  UpperLimitStiffnessUnits=N*m/deg  UpperLimitDamping=10  UpperLimitDampingUnits=N*m/(deg/s)  UpperLimitTransitionRegionWidth=0.1  UpperLimitTransitionRegionWidthUnits=deg  PositionTargetSpecify=off  PositionTargetPriority=High  PositionTargetValue=0  PositionTargetValueUnits=deg  VelocityTargetSpecify=off  VelocityTargetPriority=High  VelocityTargetValue=0  VelocityTargetValueUnits=deg/s
  q3_joint : sm_lib/Joints/Revolute Joint  JointMode=Normal  SenseConstraintForce=off  SenseConstraintForceX=off  SenseConstraintForceY=off  SenseConstraintForceZ=off  SenseConstraintTorque=off  SenseConstraintTorqueX=off  SenseConstraintTorqueY=off  SenseConstraintTorqueZ=off  SenseTotalForce=off  SenseTotalForceX=off  SenseTotalForceY=off  SenseTotalForceZ=off  SenseTotalTorque=off  SenseTotalTorqueX=off  SenseTotalTorqueY=off  SenseTotalTorqueZ=off  CompositeWrenchDir=FollowerOnBase  CompositeWrenchFrame=BaseFrame  EquilibriumPosition=0  EquilibriumPositionUnits=deg  SpringStiffness=0  SpringStiffnessUnits=N*m/deg  DampingCoefficient=b3  DampingCoefficientUnits=N*m/(deg/s)  TorqueActuationMode=InputTorque  MotionActuationMode=ComputedMotion  SensePosition=on  SenseVelocity=on  SenseAcceleration=off  SenseTorqueForce=off  SenseLowerLimitTorqueForce=off  SenseUpperLimitTorqueForce=off  LowerLimitSpecify=off  LowerLimitBound=0  LowerLimitBoundUnits=deg  LowerLimitStiffness=1e4  LowerLimitStiffnessUnits=N*m/deg  LowerLimitDamping=10  LowerLimitDampingUnits=N*m/(deg/s)  LowerLimitTransitionRegionWidth=0.1  LowerLimitTransitionRegionWidthUnits=deg  UpperLimitSpecify=off  UpperLimitBound=10  UpperLimitBoundUnits=deg  UpperLimitStiffness=1e4  UpperLimitStiffnessUnits=N*m/deg  UpperLimitDamping=10  UpperLimitDampingUnits=N*m/(deg/s)  UpperLimitTransitionRegionWidth=0.1  UpperLimitTransitionRegionWidthUnits=deg  PositionTargetSpecify=off  PositionTargetPriority=High  PositionTargetValue=0  PositionTargetValueUnits=deg  VelocityTargetSpecify=off  VelocityTargetPriority=High  VelocityTargetValue=0  VelocityTargetValueUnits=deg/s
  F : PMIOPort  Side=Left
  tau1 : PMIOPort  Port=2  Side=Left
  tau2 : PMIOPort  Port=3  Side=Left
  tau3 : PMIOPort  Port=4  Side=Left
  joiint1conn : PMIOPort  Port=5  Side=Left
  Conn6 : PMIOPort  Port=6  Side=Right
  Conn7 : PMIOPort  Port=7  Side=Right
  Conn8 : PMIOPort  Port=8  Side=Right
  d : PMIOPort  Port=9  Side=Right
  Conn10 : PMIOPort  Port=10  Side=Left
  q1 : PMIOPort  Port=11  Side=Right
  q2 : PMIOPort  Port=12  Side=Right
  q3 : PMIOPort  Port=13  Side=Right
  d_dot : PMIOPort  Port=14  Side=Right
  q1_dot : PMIOPort  Port=15  Side=Right
  q2_dot : PMIOPort  Port=16  Side=Right
  q3_dot : PMIOPort  Port=17  Side=Right
  connections:
  q3_joint/LConn1 -- T23_c/RConn1
  d_joint/RConn1 -- q1_joint/LConn1 -- RobotBase/Link1/RConn1
  Floor/World/RConn1 -- joiint1conn/RConn1 -- d_joint/LConn1
  q2_joint/RConn3 -- q2_dot/RConn1
  T34_a/RConn1 -- q3_joint/RConn1
  Link3/RConn1 -- Conn7/RConn1
  Link2/LConn1 -- q1_joint/RConn1
  T34_a/LConn1 -- Link4/LConn1
  Link4/RConn1 -- Conn8/RConn1
  Link3/LConn2 -- T23_c/LConn1
  Link2/LConn2 -- T23_a/LConn1
  T23_a/RConn1 -- q2_joint/LConn1
  T23_b/RConn1 -- q2_joint/RConn1
  Link3/LConn1 -- T23_b/LConn1
  q1_dot/RConn1 -- q1_joint/RConn3
  q1_joint/RConn2 -- q1/RConn1
  q2_joint/RConn2 -- q2/RConn1
  q3_joint/RConn2 -- q3/RConn1
  d_joint/RConn2 -- d/RConn1
  F/RConn1 -- d_joint/LConn2
  tau2/RConn1 -- q2_joint/LConn2
  tau1/RConn1 -- q1_joint/LConn2
  tau3/RConn1 -- q3_joint/LConn2
  d_dot/RConn1 -- d_joint/RConn3
  q3_joint/RConn3 -- q3_dot/RConn1
  Link2/RConn1 -- Conn6/RConn1
  Link4/LConn2 -- Conn10/RConn1

== matlab function dynamic_model_v4/Forward_Kinematics ==
  data: u input; y output
function y = Forward_Kinematics(u)

%input is joint angles
%output is x,y,z location of end effector
d= u(1);
q1= u(2);
q2= u(3);
q3= u(4);

L1= 0.2; 
L2= 0.2; 
L3= 0.3; 

c1= cos(q1); s1= sin(q1);
c2= cos(q2); s2= sin(q2);
c23= cos(q2+q3); s23= sin(q2+q3);

px= c1*(L2*c2+L3*c23);
py= s1*(L2*c2+L3*c23);
pz= L1 + d + L2*s2 +L3*s23;


y = [px,py,pz];

== matlab function dynamic_model_v4/Jacobian (J) ==
  data: u input; y output
function y = jacob(u)


d= u(1);
q1= u(2);
q2= u(3);
q3= u(4);

L1= 0.2; 
L2= 0.2; 
L3= 0.3; 

c1= cos(q1); s1= sin(q1);
c2= cos(q2); s2= sin(q2);
c23= cos(q2+q3); s23= sin(q2+q3);


J= zeros(3,4);
J(:,1)= [0;0;1];
J(:,2)= [-s1*(L2*c2+L3*c23); c1*(L2*c2+L3*c23); 0];
J(:,3)= [c1*(-L2*s2-L3*s23); s1*(-L2*s2-L3*s23); L2*c2+L3*c23];
J(:,4)= [c1*(-L3*s23); s1*(-L3*s23); L3*c23];


y = J;

== matlab function dynamic_model_v4/Control Law/M_cap ==
  settings: updateMethod=DISCRETE
  data: q input; M_mtx output; A1 input; A2 input
function M_mtx = M_cap(q, A1, A2)


%sigmoid function
function out= sigm(x)
    out= 1./ (1 + exp(x));
end


%compute M
layer1= sigm(A2*q);
M= A1*layer1;

%convert to mtx
M_mtx= [M(1), M(2), M(3);
    M(4), M(5), M(6);
    M(7), M(8), M(9)];


end

== matlab function dynamic_model_v4/Control Law/C_cap ==
  data: q input; C_mtx output; q_dot input; B1 input; B2 input
function C_mtx = C_cap(q, q_dot, B1, B2)



%sigmoid function
function out= sigm(x)
    out= 1./ (1 + exp(x));
end

%compute C
layer1= sigm(B2*[q;q_dot]);
C= B1*layer1;

%convert to mtx
C_mtx= [C(1), C(2), C(3);
    C(4), C(5), C(6);
    C(7), C(8), C(9)];

end

== matlab function dynamic_model_v4/Control Law/H_cap ==
  data: q input; H_mtx output; q_dot input; C1 input; C2 input
function H_mtx = H_cap(q, q_dot, C1, C2)

%sigmoid function
function out= sigm(x)
    out= 1./ (1 + exp(x));
end

%compute H
layer1= sigm(C2*[q;q_dot]);
H= C1*layer1;

%convert to mtx
H_mtx= [H(1);
    H(2);
    H(3)];


end

== matlab function dynamic_model_v4/Control Law/NN Params Adpatation Rules ==
  settings: updateMethod=DISCRETE
  data: q input; q_dot input; A1_out output; s input; xr_2dot input; A1 input; A2 input; A2_out output; B1 input; B2 input; C1 input; C2 input; B1_out output; B2_out output; C1_out output; C2_out output
function [A1_out, A2_out, B1_out, B2_out, C1_out, C2_out] = NN_adaptation(q, q_dot, s, xr_2dot, A1, A2, B1, B2, C1, C2)


%sigmoid function
function out= sigm(x)
    out= 1./ (1 + exp(x));
end

%Derivative of sigmoid
function out= sigm_dot(x)
    out= exp(-x)./(exp(-x) + 1).^2;
end


%Adaption params
k= 5; %kappa %default: 5
g_M= ones(9,1); %gamma M
g_C= 1; %gamma C
g_H= 1; %gamma H

%Adaptation rules 
% A1_dot= -k*(sqrt(sum(s.^2)))*A1 - g_M*(sigm(A2*q) + (sigm_dot(A2*q).*(A2*q)))'.*(xr_2dot'*s);
% A2_dot= -k*(sqrt(sum(s.^2)))*A2;
% B1_dot= -k*(sqrt(sum(s.^2)))*B1;
% B2_dot= -k*(sqrt(sum(s.^2)))*B2;
% C1_dot= -k*(sqrt(sum(s.^2)))*C1;
% C2_dot= -k*(sqrt(sum(s.^2)))*C2;


%Adaptation rules Simplified
A1_dot= -k*(sqrt(sum(s.^2)))*A1;
A2_dot= -k*(sqrt(sum(s.^2)))*A2;
B1_dot= -k*(sqrt(sum(s.^2)))*B1;
B2_dot= -k*(sqrt(sum(s.^2)))*B2;
C1_dot= -k*(sqrt(sum(s.^2)))*C1;
C2_dot= -k*(sqrt(sum(s.^2)))*C2;


%Update NN params
A1_out= A1 + A1_dot;
A2_out= A2 + A2_dot;
B1_out= B1 + B1_dot;
B2_out= B2 + B2_dot;
C1_out= C1 + C1_dot;
C2_out= C2 + C2_dot;



end
